simulink model "updown_counter_withhold"  (R2025a)
settings: Solver=FixedStepDiscrete  StartTime=0.0  StopTime=100  FixedStep=1  RelTol=1e-3
settings Model: Creator=Admin  LastModifiedBy=DELL PC

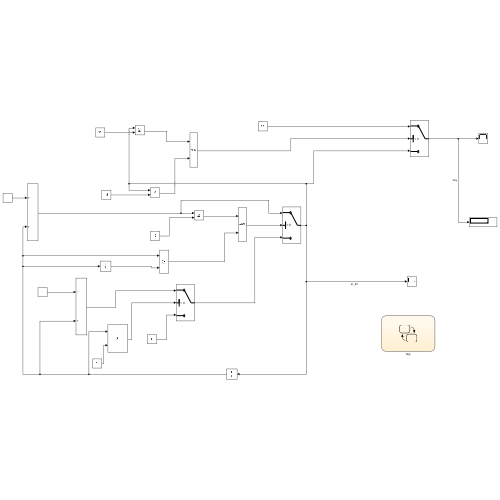
[thumbnail: Simulink's stored preview of the top-level diagram]
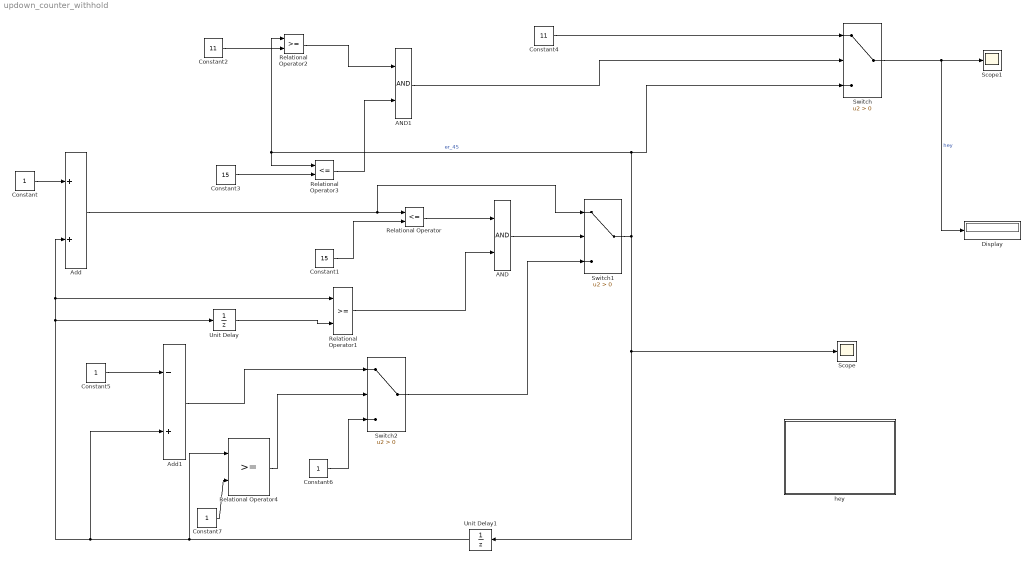
== system updown_counter_withhold ==
  AND : Logic  AllPortsSameDT=off  OutDataTypeStr=boolean
  AND1 : Logic  AllPortsSameDT=off  OutDataTypeStr=boolean
  Add : Sum
  Add1 : Sum  Inputs=-+
  Constant{,5..7} (4 alike) : Constant
  Constant1 : Constant  Value=15
  Constant2 : Constant  Value=11
  Constant3 : Constant  Value=15
  Constant4 : Constant  Value=11
  Display : Display
  Relational Operator : RelationalOperator  Operator=<=  OutDataTypeStr=boolean  RndMeth=Simplest  InputSameDT=off
  Relational Operator1 : RelationalOperator  OutDataTypeStr=boolean  RndMeth=Simplest  InputSameDT=off
  Relational Operator2 : RelationalOperator  OutDataTypeStr=boolean  RndMeth=Simplest  InputSameDT=off
  Relational Operator3 : RelationalOperator  Operator=<=  OutDataTypeStr=boolean  RndMeth=Simplest  InputSameDT=off
  Relational Operator4 : RelationalOperator  OutDataTypeStr=boolean  RndMeth=Simplest  InputSameDT=off
  Scope : Scope
  Scope1 : Scope
      settings: ActiveDisplayYMinimum=-2.5  ActiveDisplayYMaximum=12.5
  Switch : Switch  Criteria=u2 > Threshold  SaturateOnIntegerOverflow=off  InputSameDT=off
  Switch1 : Switch  Criteria=u2 > Threshold  SaturateOnIntegerOverflow=off  InputSameDT=off
  Switch2 : Switch  Criteria=u2 > Threshold  SaturateOnIntegerOverflow=off  InputSameDT=off
  Unit Delay : UnitDelay  SampleTime=-1  HasFrameUpgradeWarning=on
  Unit Delay1 : UnitDelay  SampleTime=-1  HasFrameUpgradeWarning=on
  hey : Stateflow chart  TreatAsAtomicUnit=on
  wires:
  Constant3/1 -> Relational Operator3/2
  Add1/1 -> Switch2/1
  AND1/1 -> Switch/2
  Constant/1 -> Add/1
  Relational Operator2/1 -> AND1/1
  Relational Operator4/1 -> Switch2/2
  Constant4/1 -> Switch/1
  Relational Operator3/1 -> AND1/2
  Constant6/1 -> Switch2/3
  Unit Delay/1 -> Relational Operator1/2
  Relational Operator1/1 -> AND/2
  Constant5/1 -> Add1/1
  Unit Delay1/1 -> Add1/2, Unit Delay/1, Add/2, Relational Operator1/1, Relational Operator4/1
  Relational Operator/1 -> AND/1
  AND/1 -> Switch1/2
  Constant2/1 -> Relational Operator2/2
  Constant7/1 -> Relational Operator4/2
  Constant1/1 -> Relational Operator/2
  Switch2/1 -> Switch1/3
  Add/1 -> Switch1/1, Relational Operator/1
  Switch/1 -> Display/1, Scope1/1  "hey"
  Switch1/1 -> Scope/1, Unit Delay1/1, Switch/3, Relational Operator3/1, Relational Operator2/1  "er_45"

== stateflow chart updown_counter_withhold/hey ==
